simulink model "VIPR4sStEnCtrl"  (R2018b)
settings: Solver=FixedStepDiscrete  StartTime=0.0  StopTime=10.0  FixedStep=0.01  RelTol=1e-3
undefined symbols (not defined in the file or in its folder): data, KeSMSw4SSecRwRtStLgrstUpwdDnwdOpenPos1_Val, SecRwRtStBkReclnEn_Clear, SecRwRtStBkReclnEn_Set, SecRwRtStFtrstEn_Clear, SecRwRtStFtrstEn_Set, SecRwRtStFwdBkwdEn_Clear, SecRwRtStFwdBkwdEn_Set, SecRwRtStHdrstFwdBkwdEn_Clear, SecRwRtStHdrstFwdBkwdEn_Set, SecRwRtStHdrstUpwdDnwdEn_Clear, SecRwRtStHdrstUpwdDnwdEn_Set, SecRwRtStLgrstInwdOtwdEn_Clear, SecRwRtStLgrstInwdOtwdEn_Set, SecRwRtStLgrstUpwdDnwdEn_Clear, SecRwRtStLgrstUpwdDnwdEn_Set
libraries: simulink x16
settings Model: Creator=sn2xws  LastModifiedBy=sn2xws
settings Model: ModifiedHistory=|
  | 2023.11.16  V2.3.0 Issue 566045 全躺，vip，腿托打开增加前后位置
  | 2023.12.22
settings DataIOCC: SaveFormat=StructureWithTime
settings OptimizationCC: DefaultParameterBehavior=Inlined  EnhancedBackFolding=on  PassReuseOutputArgsAs=Individual arguments  ZeroExternalMemoryAtStartup=off  ZeroInternalMemoryAtStartup=off  OptimizeBlockOrder=speed  DifferentSizesBufferReuse=on  OptimizationCustomize=off
settings DebuggingCC: ParameterTunabilityLossMsg=error
settings SFSimCC: MATLABDynamicMemAlloc=off
settings RTWCC: SystemTargetFile=autosar.tlc  GenCodeOnly=on  TemplateMakefile=ert_default_tmf  Description=AUTOSAR  GenerateReport=on  IncludeHyperlinkInReport=on  LaunchReport=on  GenerateTraceInfo=on  GenerateTraceReport=on  GenerateTraceReportSl=on  GenerateTraceReportSf=on  GenerateTraceReportEml=on  GenerateCodeMetricsReport=on
settings CodeAppCC: ForceParamTrailComments=on  IgnoreCustomStorageClasses=off  OperatorAnnotations=on  SimulinkDataObjDesc=on  SFDataObjDesc=on  InsertBlockDesc=on
settings STFCustomTargetCC: TargetLangStandard=C99 (ISO)  MultiwordLength=256  ParMdlRefBuildCompliant=on  CompOptLevelCompliant=on  IncludeMdlTerminateFcn=off  CombineOutputUpdateFcns=on  SuppressErrorStatus=on  ERTCustomFileBanners=on  SupportNonFinite=off  SupportComplex=off  SupportContinuousTime=off  SupportNonInlinedSFcns=off  RemoveResetFunc=on  MATLABClassNameForMDSCustomization=Simulink.SoftwareTarget.ERTCustomization  AutosarCompliant=on  UseToolchainInfoCompliant=on  LookupTableObjectStructAxisOrder=2,1,3,4,...  LUTObjectStructOrderEvenSpacing=Size,Table,Breakpoints  SystemTargetFile=autosar.tlc
settings ERTTargetCC: TargetLangStandard=C99 (ISO)  ConcurrentExecutionCompliant=off  IncludeMdlTerminateFcn=off  SuppressErrorStatus=on  SupportNonFinite=off  SupportComplex=off  ModelStepFunctionPrototypeControlCompliant=off  CPPClassGenCompliant=off  AutosarCompliant=on  LookupTableObjectStructAxisOrder=2,1,3,4,...  LUTObjectStructOrderEvenSpacing=Size,Table,Breakpoints  InlinedParameterPlacement=NonHierarchical  ERTCustomFileTemplate=example_file_process.tlc  ERTFilePackagingFormat=Compact

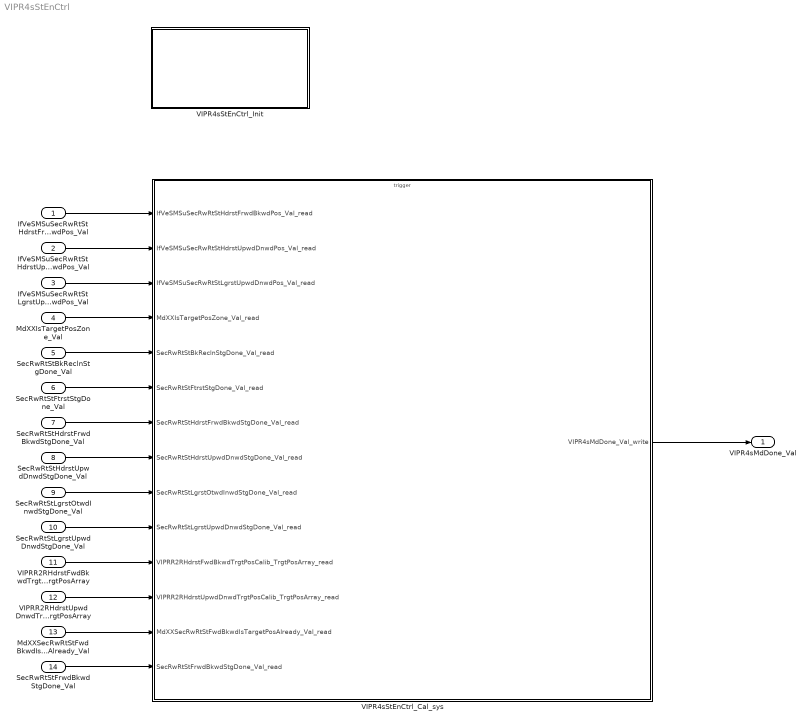
== system VIPR4sStEnCtrl ==
  IfVeSMSuSecRwRtStHdrstFrwdBkwdPos_Val : Inport  OutDataTypeStr=uint16  PortDimensions=1
  IfVeSMSuSecRwRtStHdrstUpwdDnwdPos_Val : Inport  Port=2  OutDataTypeStr=uint16  PortDimensions=1
  IfVeSMSuSecRwRtStLgrstUpwdDnwdPos_Val : Inport  Port=3  OutDataTypeStr=uint16  PortDimensions=1
  MdXXIsTargetPosZone_Val : Inport  Port=4  OutDataTypeStr=uint32  PortDimensions=1
  SecRwRtStBkReclnStgDone_Val : Inport  Port=5  OutDataTypeStr=boolean  PortDimensions=1
  SecRwRtStFtrstStgDone_Val : Inport  Port=6  OutDataTypeStr=boolean  PortDimensions=1
  SecRwRtStHdrstFrwdBkwdStgDone_Val : Inport  Port=7  OutDataTypeStr=boolean  PortDimensions=1
  SecRwRtStHdrstUpwdDnwdStgDone_Val : Inport  Port=8  OutDataTypeStr=boolean  PortDimensions=1
  SecRwRtStLgrstOtwdInwdStgDone_Val : Inport  Port=9  OutDataTypeStr=boolean  PortDimensions=1
  SecRwRtStLgrstUpwdDnwdStgDone_Val : Inport  Port=10  OutDataTypeStr=boolean  PortDimensions=1
  VIPRR2RHdrstFwdBkwdTrgtPosCalib_TrgtPosArray : Inport  Description=|  Port=11  OutDataTypeStr=uint16  PortDimensions=3
      | 0:Pos
      | 1:Max
      | 2:Min
  VIPRR2RHdrstUpwdDnwdTrgtPosCalib_TrgtPosArray : Inport  Description=|  Port=12  OutDataTypeStr=uint16  PortDimensions=3
      | 0:Pos
      | 1:Max
      | 2:Min
  MdXXSecRwRtStFwdBkwdIsTargetPosAlready_Val : Inport  Port=13  OutDataTypeStr=uint32  PortDimensions=1
  SecRwRtStFrwdBkwdStgDone_Val : Inport  Port=14  OutDataTypeStr=boolean  PortDimensions=1
  VIPR4sStEnCtrl_Cal_sys : Subsystem
  VIPR4sStEnCtrl_Init : Subsystem
  VIPR4sMdDone_Val : Outport  OutDataTypeStr=uint8  PortDimensions=1
  wires:
  IfVeSMSuSecRwRtStHdrstFrwdBkwdPos_Val/1 -> VIPR4sStEnCtrl_Cal_sys/1(IfVeSMSuSecRwRtStHdrstFrwdBkwdPos_Val_read)
  IfVeSMSuSecRwRtStHdrstUpwdDnwdPos_Val/1 -> VIPR4sStEnCtrl_Cal_sys/2(IfVeSMSuSecRwRtStHdrstUpwdDnwdPos_Val_read)
  IfVeSMSuSecRwRtStLgrstUpwdDnwdPos_Val/1 -> VIPR4sStEnCtrl_Cal_sys/3(IfVeSMSuSecRwRtStLgrstUpwdDnwdPos_Val_read)
  MdXXIsTargetPosZone_Val/1 -> VIPR4sStEnCtrl_Cal_sys/4(MdXXIsTargetPosZone_Val_read)
  SecRwRtStBkReclnStgDone_Val/1 -> VIPR4sStEnCtrl_Cal_sys/5(SecRwRtStBkReclnStgDone_Val_read)
  SecRwRtStFtrstStgDone_Val/1 -> VIPR4sStEnCtrl_Cal_sys/6(SecRwRtStFtrstStgDone_Val_read)
  SecRwRtStHdrstFrwdBkwdStgDone_Val/1 -> VIPR4sStEnCtrl_Cal_sys/7(SecRwRtStHdrstFrwdBkwdStgDone_Val_read)
  SecRwRtStHdrstUpwdDnwdStgDone_Val/1 -> VIPR4sStEnCtrl_Cal_sys/8(SecRwRtStHdrstUpwdDnwdStgDone_Val_read)
  SecRwRtStLgrstOtwdInwdStgDone_Val/1 -> VIPR4sStEnCtrl_Cal_sys/9(SecRwRtStLgrstOtwdInwdStgDone_Val_read)
  SecRwRtStLgrstUpwdDnwdStgDone_Val/1 -> VIPR4sStEnCtrl_Cal_sys/10(SecRwRtStLgrstUpwdDnwdStgDone_Val_read)
  VIPRR2RHdrstFwdBkwdTrgtPosCalib_TrgtPosArray/1 -> VIPR4sStEnCtrl_Cal_sys/11(VIPRR2RHdrstFwdBkwdTrgtPosCalib_TrgtPosArray_read)
  VIPRR2RHdrstUpwdDnwdTrgtPosCalib_TrgtPosArray/1 -> VIPR4sStEnCtrl_Cal_sys/12(VIPRR2RHdrstUpwdDnwdTrgtPosCalib_TrgtPosArray_read)
  VIPR4sStEnCtrl_Cal_sys/1(VIPR4sMdDone_Val_write) -> VIPR4sMdDone_Val/1
  MdXXSecRwRtStFwdBkwdIsTargetPosAlready_Val/1 -> VIPR4sStEnCtrl_Cal_sys/13(MdXXSecRwRtStFwdBkwdIsTargetPosAlready_Val_read)
  SecRwRtStFrwdBkwdStgDone_Val/1 -> VIPR4sStEnCtrl_Cal_sys/14(SecRwRtStFrwdBkwdStgDone_Val_read)

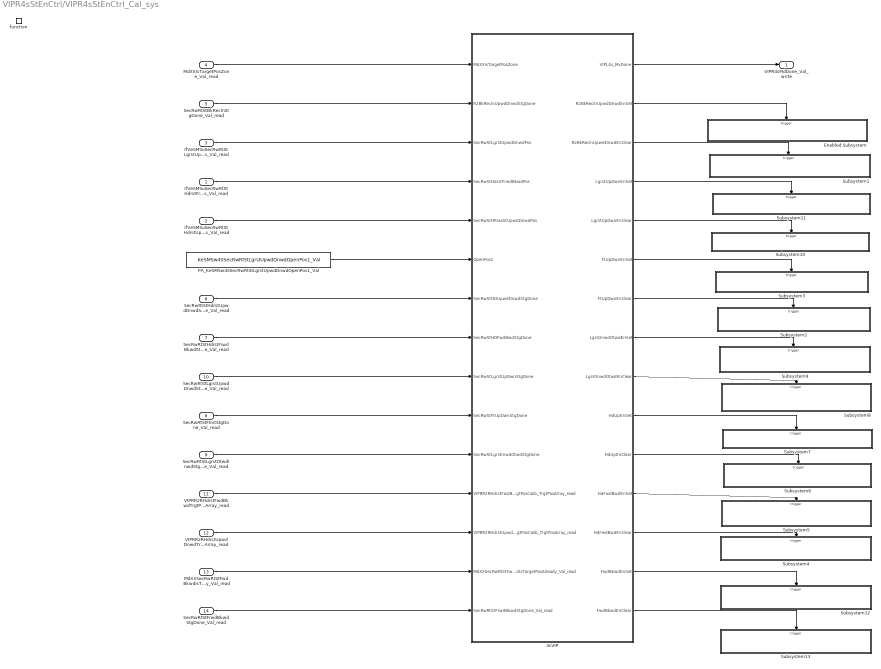
== system VIPR4sStEnCtrl/VIPR4sStEnCtrl_Cal_sys ==
  IfVeSMSuSecRwRtStHdrstFrwdBkwdPos_Val_read : Inport
  IfVeSMSuSecRwRtStHdrstUpwdDnwdPos_Val_read : Inport  Port=2
  IfVeSMSuSecRwRtStLgrstUpwdDnwdPos_Val_read : Inport  Port=3
  MdXXIsTargetPosZone_Val_read : Inport  Port=4
  SecRwRtStBkReclnStgDone_Val_read : Inport  Port=5
  SecRwRtStFtrstStgDone_Val_read : Inport  Port=6
  SecRwRtStHdrstFrwdBkwdStgDone_Val_read : Inport  Port=7
  SecRwRtStHdrstUpwdDnwdStgDone_Val_read : Inport  Port=8
  SecRwRtStLgrstOtwdInwdStgDone_Val_read : Inport  Port=9
  SecRwRtStLgrstUpwdDnwdStgDone_Val_read : Inport  Port=10
  VIPRR2RHdrstFwdBkwdTrgtPosCalib_TrgtPosArray_read : Inport  Port=11
  VIPRR2RHdrstUpwdDnwdTrgtPosCalib_TrgtPosArray_read : Inport  Port=12
  MdXXSecRwRtStFwdBkwdIsTargetPosAlready_Val_read : Inport  Port=13
  SecRwRtStFrwdBkwdStgDone_Val_read : Inport  Port=14
  function : TriggerPort  TriggerType=function-call  IsSimulinkFunction=on  FunctionName=VIPR4sStEnCtrl_Cal  VariantControl=(inherit)
  4sVIP : Subsystem
  Enabled Subsystem : Subsystem  TreatAsAtomicUnit=on
  PA_KeSMSw4SSecRwRtStLgrstUpwdDnwdOpenPos1_Val : Constant  Value=KeSMSw4SSecRwRtStLgrstUpwdDnwdOpenPos1_Val
  Subsystem1 : Subsystem
  Subsystem10 : Subsystem
  Subsystem11 : Subsystem
  Subsystem12 : Subsystem
  Subsystem13 : Subsystem
  Subsystem2 : Subsystem
  Subsystem3 : Subsystem
  Subsystem4 : Subsystem
  Subsystem5 : Subsystem
  Subsystem6 : Subsystem
  Subsystem7 : Subsystem
  Subsystem8 : Subsystem
  Subsystem9 : Subsystem
  VIPR4sMdDone_Val_write : Outport
      settings: EnsureOutportIsVirtual=on
  wires:
  IfVeSMSuSecRwRtStHdrstFrwdBkwdPos_Val_read/1 -> 4sVIP/4(SecRwStHdrstFrwdBkwdPos)
  IfVeSMSuSecRwRtStHdrstUpwdDnwdPos_Val_read/1 -> 4sVIP/5(SecRwStHPassStUpwdDnwdPos)
  VIPRR2RHdrstFwdBkwdTrgtPosCalib_TrgtPosArray_read/1 -> 4sVIP/12(VIPRR2RHdrstFwdBkwdTrgtPosCalib_TrgtPosArray_read)
  VIPRR2RHdrstUpwdDnwdTrgtPosCalib_TrgtPosArray_read/1 -> 4sVIP/13(VIPRR2RHdrstUpwdDnwdTrgtPosCalib_TrgtPosArray_read)
  4sVIP/1(VIPL4s_MvDone) -> VIPR4sMdDone_Val_write/1
  PA_KeSMSw4SSecRwRtStLgrstUpwdDnwdOpenPos1_Val/1 -> 4sVIP/6(OpenPos1)
  MdXXIsTargetPosZone_Val_read/1 -> 4sVIP/1(MdXXIsTargetPosZone)
  SecRwRtStBkReclnStgDone_Val_read/1 -> 4sVIP/2(R2BkReclnUpwdDnwdStgDone)
  IfVeSMSuSecRwRtStLgrstUpwdDnwdPos_Val_read/1 -> 4sVIP/3(SecRwStLgrstUpwdDnwdPos)
  SecRwRtStHdrstUpwdDnwdStgDone_Val_read/1 -> 4sVIP/7(SecRwStHDUpwdDnwdStgDone)
  SecRwRtStHdrstFrwdBkwdStgDone_Val_read/1 -> 4sVIP/8(SecRwStHDFwdBwdStgDone)
  SecRwRtStLgrstUpwdDnwdStgDone_Val_read/1 -> 4sVIP/9(SecRwStLgrstUpDwnStgDone)
  SecRwRtStLgrstOtwdInwdStgDone_Val_read/1 -> 4sVIP/11(SecRwStLgrstInwdOtwdStgDone)
  SecRwRtStFtrstStgDone_Val_read/1 -> 4sVIP/10(SecRwStFtUpDwnStgDone)
  4sVIP/13(HdFwdBwdEnClear) -> Subsystem4/Trigger
  4sVIP/2(R2BkReclnUpwdDnwdEnSet) -> Enabled Subsystem/Trigger
  4sVIP/3(R2BkReclnUpwdDnwdEnClear) -> Subsystem1/Trigger
  4sVIP/5(LgrstUpDwnEnClear) -> Subsystem10/Trigger
  4sVIP/11(HdUpEnClear) -> Subsystem6/Trigger
  4sVIP/10(HdUpEnSet) -> Subsystem7/Trigger
  4sVIP/8(LgrstInwdOtwdEnSet) -> Subsystem9/Trigger
  4sVIP/9(LgrstInwdOtwdEnClear) -> Subsystem8/Trigger
  4sVIP/6(FtUpDwnEnSet) -> Subsystem3/Trigger
  4sVIP/7(FtUpDwnEnClear) -> Subsystem2/Trigger
  4sVIP/12(HdFwdBwdEnSet) -> Subsystem5/Trigger
  4sVIP/4(LgrstUpDwnEnSet) -> Subsystem11/Trigger
  MdXXSecRwRtStFwdBkwdIsTargetPosAlready_Val_read/1 -> 4sVIP/14(MdXXSecRwRtStFwdBkwdIsTargetPosAlready_Val_read)
  SecRwRtStFrwdBkwdStgDone_Val_read/1 -> 4sVIP/15(SecRwRtStFrwdBkwdStgDone_Val_read)
  4sVIP/14(FwdBkwdEnSet) -> Subsystem12/Trigger
  4sVIP/15(FwdBkwdEnClear) -> Subsystem13/Trigger

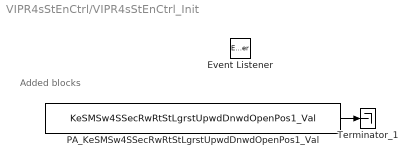
== system VIPR4sStEnCtrl/VIPR4sStEnCtrl_Init ==
  note: Added blocks
  Event Listener : EventListener  EventName=reset
  PA_KeSMSw4SSecRwRtStLgrstUpwdDnwdOpenPos1_Val : Constant  Value=KeSMSw4SSecRwRtStLgrstUpwdDnwdOpenPos1_Val
  Terminator_1 : Terminator
  wires:
  PA_KeSMSw4SSecRwRtStLgrstUpwdDnwdOpenPos1_Val/1 -> Terminator_1/1

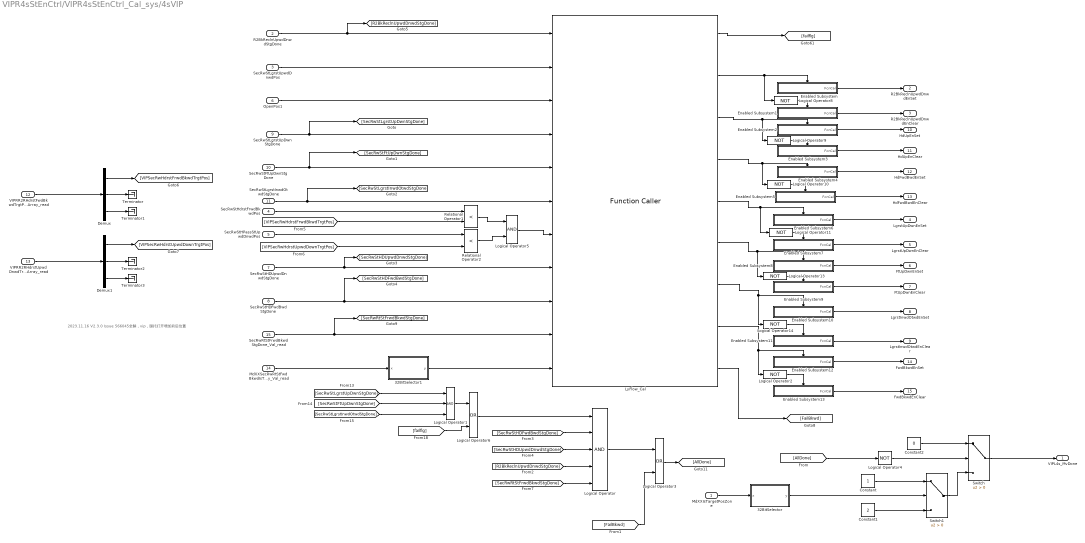
== system VIPR4sStEnCtrl/VIPR4sStEnCtrl_Cal_sys/4sVIP ==
  note: 2023.11.16 V2.3.0 Issue 566045 全躺，vip，腿托打开增加前后位置
  MdXXIsTargetPosZone : Inport
  R2BkReclnUpwdDnwdStgDone : Inport  Port=2
  SecRwStLgrstUpwdDnwdPos : Inport  Port=3
  SecRwStHdrstFrwdBkwdPos : Inport  Port=4
  SecRwStHPassStUpwdDnwdPos : Inport  Port=5
  OpenPos1 : Inport  Port=6
  SecRwStHDUpwdDnwdStgDone : Inport  Port=7
  SecRwStHDFwdBwdStgDone : Inport  Port=8
  SecRwStLgrstUpDwnStgDone : Inport  Port=9
  SecRwStFtUpDwnStgDone : Inport  Port=10
  SecRwStLgrstInwdOtwdStgDone : Inport  Port=11
  VIPRR2RHdrstFwdBkwdTrgtPosCalib_TrgtPosArray_read : Inport  Port=12
  VIPRR2RHdrstUpwdDnwdTrgtPosCalib_TrgtPosArray_read : Inport  Port=13
  MdXXSecRwRtStFwdBkwdIsTargetPosAlready_Val_read : Inport  Port=14
  SecRwRtStFrwdBkwdStgDone_Val_read : Inport  Port=15
  32BitSelector : Subsystem  mask(32 Bit Selector){BitNum=11}
      mask prompts: BitNum "Select Bit Number"
      mask help: Allows selection of a particular bit (0-31) out of a packed word up to 32 bits long. Output will be true if the bit number selected via the mask parameter is equal to one.
      mask TypeOptions BitNum: 0 | 1 | 2 | 3 | 4 | 5 | 6 | 7 | 8 | 9 | 10 | 11 | 12 | 13 | 14 | 15 | 16 | 17 | 18 | 19 | 20 | 21 | 22 | 23 | 24 | 25 | 26 | 27 | 28 | 29 | 30 | 31
      mask Display:
      | text(0.5, 0.8,'BIT','horizontalAlignment','center')
      | text(0.5, 0.5,'SELECTOR','horizontalAlignment','center')
      | text(0.5, 0.2,['-- Bit ',char(get_param(gcb,'BitNum')),' --'],'horizontalAlignment','center')
  32BitSelector1 : Subsystem  mask(32 Bit Selector){BitNum=11}
      mask prompts: BitNum "Select Bit Number"
      mask help: Allows selection of a particular bit (0-31) out of a packed word up to 32 bits long. Output will be true if the bit number selected via the mask parameter is equal to one.
      mask TypeOptions BitNum: 0 | 1 | 2 | 3 | 4 | 5 | 6 | 7 | 8 | 9 | 10 | 11 | 12 | 13 | 14 | 15 | 16 | 17 | 18 | 19 | 20 | 21 | 22 | 23 | 24 | 25 | 26 | 27 | 28 | 29 | 30 | 31
      mask Display:
      | text(0.5, 0.8,'BIT','horizontalAlignment','center')
      | text(0.5, 0.5,'SELECTOR','horizontalAlignment','center')
      | text(0.5, 0.2,['-- Bit ',char(get_param(gcb,'BitNum')),' --'],'horizontalAlignment','center')
  Constant : Constant  OutDataTypeStr=uint8
  Constant1 : Constant  Value=2  OutDataTypeStr=uint8
  Constant2 : Constant  Value=0  OutDataTypeStr=uint8
  Demux : Demux  Outputs=3
  Demux1 : Demux  Outputs=3
  Enabled Subsystem : Subsystem  TreatAsAtomicUnit=on
  Enabled Subsystem1 : Subsystem  TreatAsAtomicUnit=on
  Enabled Subsystem10 : Subsystem  TreatAsAtomicUnit=on
  Enabled Subsystem11 : Subsystem  TreatAsAtomicUnit=on
  Enabled Subsystem12 : Subsystem  TreatAsAtomicUnit=on
  Enabled Subsystem13 : Subsystem  TreatAsAtomicUnit=on
  Enabled Subsystem2 : Subsystem  TreatAsAtomicUnit=on
  Enabled Subsystem3 : Subsystem  TreatAsAtomicUnit=on
  Enabled Subsystem4 : Subsystem  TreatAsAtomicUnit=on
  Enabled Subsystem5 : Subsystem  TreatAsAtomicUnit=on
  Enabled Subsystem6 : Subsystem  TreatAsAtomicUnit=on
  Enabled Subsystem7 : Subsystem  TreatAsAtomicUnit=on
  Enabled Subsystem8 : Subsystem  TreatAsAtomicUnit=on
  Enabled Subsystem9 : Subsystem  TreatAsAtomicUnit=on
  Logical Operator : Logic  Inputs=5  AllPortsSameDT=off  OutDataTypeStr=boolean
  Logical Operator1 : Logic  Inputs=3  AllPortsSameDT=off  OutDataTypeStr=boolean
  Logical Operator{2,4,8..11,13..14} (8 alike) : Logic  Operator=NOT  AllPortsSameDT=off  OutDataTypeStr=boolean
  Logical Operator3 : Logic  Operator=OR  AllPortsSameDT=off  OutDataTypeStr=boolean
  Logical Operator5 : Logic  AllPortsSameDT=off  OutDataTypeStr=boolean
  Logical Operator6 : Logic  Operator=OR  AllPortsSameDT=off  OutDataTypeStr=boolean
  LyFlow_Cal : FunctionCaller  FunctionPrototype=[Failflg,BkReclnEn,HdrstUpwdEn,HdrstFrwdEn,LgrstUpwdDnwdEn,FtrstEn,LgrstInwdOtwdEn,FwdBkwdEn,FailBkwd] = LyFlow_Cal(BkReclnStgDone,LgrstUpwdDnwdPos,LgrstUpwdDnwdOpenPos1,LgrstUpwdStgDone,FtrstStgDone,LgrstInwdStgDone,Chkhdflg,HdrstUpwdDnwdStgDone,HdrstFrwdBkwdStgDone,FwdBkwdStgDone,FwdBkwdIsPosAlready)  InputArgumentSpecifications=boolean(true), uint16(1), uint16(1), boolean(true), boolean(true), boolean(true), boolean(true), boolean(true), boolean(true), boolean(true), boolean(true)  OutputArgumentSpecifications=boolean(true), boolean(true), boolean(true), boolean(true), boolean(true), boolean(true), boolean(true), boolean(true), boolean(true)
  Relational Operator1 : RelationalOperator  Operator=<  OutDataTypeStr=boolean  RndMeth=Simplest
  Relational Operator2 : RelationalOperator  Operator=<  OutDataTypeStr=boolean  RndMeth=Simplest
  Switch : Switch  Criteria=u2 > Threshold
  Switch1 : Switch  Criteria=u2 > Threshold
  Terminator{,1..3} (4 alike) : Terminator
  VIPL4s_MvDone : Outport
  R2BkReclnUpwdDnwdEnSet : Outport  Port=2
  R2BkReclnUpwdDnwdEnClear : Outport  Port=3
  LgrstUpDwnEnSet : Outport  Port=4
  LgrstUpDwnEnClear : Outport  Port=5
  FtUpDwnEnSet : Outport  Port=6
  FtUpDwnEnClear : Outport  Port=7
  LgrstInwdOtwdEnSet : Outport  Port=8
  LgrstInwdOtwdEnClear : Outport  Port=9
  HdUpEnSet : Outport  Port=10
  HdUpEnClear : Outport  Port=11
  HdFwdBwdEnSet : Outport  Port=12
  HdFwdBwdEnClear : Outport  Port=13
  FwdBkwdEnSet : Outport  Port=14
  FwdBkwdEnClear : Outport  Port=15
  wires:
  [VIPSecRwHdrstUpwdDownTrgtPos] -> Relational Operator2/2
  [R2BkReclnUpwdDnwdStgDone] -> Logical Operator/4
  [SecRwStFtUpDwnStgDone] -> Logical Operator1/2
  [SecRwStHDFwdBwdStgDone] -> Logical Operator/2
  SecRwStHDFwdBwdStgDone/1 -> [SecRwStHDFwdBwdStgDone], LyFlow_Cal/9
  Logical Operator5/1 -> LyFlow_Cal/7
  OpenPos1/1 -> LyFlow_Cal/3
  SecRwStLgrstInwdOtwdStgDone/1 -> [SecRwStLgrstInwdOtwdStgDone], LyFlow_Cal/6
  [failflg] -> Logical Operator6/2
  SecRwStHdrstFrwdBkwdPos/1 -> Relational Operator1/1
  Relational Operator2/1 -> Logical Operator5/2
  SecRwStFtUpDwnStgDone/1 -> LyFlow_Cal/5, [SecRwStFtUpDwnStgDone]
  [SecRwStLgrstInwdOtwdStgDone] -> Logical Operator1/3
  SecRwStHPassStUpwdDnwdPos/1 -> Relational Operator2/1
  [SecRwStLgrstUpDwnStgDone] -> Logical Operator1/1
  Logical Operator1/1 -> Logical Operator6/1
  Logical Operator6/1 -> Logical Operator/1
  [SecRwStHDUpwdDnwdStgDone] -> Logical Operator/3
  MdXXIsTargetPosZone/1 -> 32BitSelector/1(x)
  Relational Operator1/1 -> Logical Operator5/1
  SecRwStHDUpwdDnwdStgDone/1 -> [SecRwStHDUpwdDnwdStgDone], LyFlow_Cal/8
  LyFlow_Cal/1 -> [failflg]
  SecRwStLgrstUpwdDnwdPos/1 -> LyFlow_Cal/2
  R2BkReclnUpwdDnwdStgDone/1 -> [R2BkReclnUpwdDnwdStgDone], LyFlow_Cal/1
  [VIPSecRwHdrstFrwdBkwdTrgtPos] -> Relational Operator1/2
  SecRwStLgrstUpDwnStgDone/1 -> [SecRwStLgrstUpDwnStgDone], LyFlow_Cal/4
  Switch/1 -> VIPL4s_MvDone/1
  Switch1/1 -> Switch/3
  Enabled Subsystem5/1(FcnCal) -> HdFwdBwdEnClear/1
  Enabled Subsystem6/1(FcnCal) -> LgrstUpDwnEnSet/1
  Logical Operator11/1 -> Enabled Subsystem7/Enable
  Enabled Subsystem/1(FcnCal) -> R2BkReclnUpwdDnwdEnSet/1
  LyFlow_Cal/7 -> Logical Operator14/1, Enabled Subsystem10/Enable
  Enabled Subsystem3/1(FcnCal) -> HdUpEnClear/1
  Enabled Subsystem1/1(FcnCal) -> R2BkReclnUpwdDnwdEnClear/1
  Logical Operator9/1 -> Enabled Subsystem3/Enable
  Logical Operator14/1 -> Enabled Subsystem11/Enable
  Logical Operator10/1 -> Enabled Subsystem5/Enable
  LyFlow_Cal/2 -> Logical Operator8/1, Enabled Subsystem/Enable
  LyFlow_Cal/6 -> Logical Operator13/1, Enabled Subsystem8/Enable
  Enabled Subsystem10/1(FcnCal) -> LgrstInwdOtwdEnSet/1
  Logical Operator13/1 -> Enabled Subsystem9/Enable
  Enabled Subsystem11/1(FcnCal) -> LgrstInwdOtwdEnClear/1
  Logical Operator8/1 -> Enabled Subsystem1/Enable
  Enabled Subsystem2/1(FcnCal) -> HdUpEnSet/1
  LyFlow_Cal/3 -> Logical Operator9/1, Enabled Subsystem2/Enable
  Enabled Subsystem8/1(FcnCal) -> FtUpDwnEnSet/1
  Enabled Subsystem7/1(FcnCal) -> LgrstUpDwnEnClear/1
  LyFlow_Cal/5 -> Logical Operator11/1, Enabled Subsystem6/Enable
  Enabled Subsystem4/1(FcnCal) -> HdFwdBwdEnSet/1
  LyFlow_Cal/4 -> Logical Operator10/1, Enabled Subsystem4/Enable
  Enabled Subsystem9/1(FcnCal) -> FtUpDwnEnClear/1
  VIPRR2RHdrstFwdBkwdTrgtPosCalib_TrgtPosArray_read/1 -> Demux/1
  Demux/1 -> [VIPSecRwHdrstFrwdBkwdTrgtPos]
  Demux/2 -> Terminator/1
  Demux/3 -> Terminator1/1
  Demux1/3 -> Terminator3/1
  Demux1/2 -> Terminator2/1
  Demux1/1 -> [VIPSecRwHdrstUpwdDownTrgtPos]
  VIPRR2RHdrstUpwdDnwdTrgtPosCalib_TrgtPosArray_read/1 -> Demux1/1
  Constant2/1 -> Switch/1
  Constant1/1 -> Switch1/3
  Constant/1 -> Switch1/1
  [AllDone] -> Logical Operator4/1
  Logical Operator4/1 -> Switch/2
  32BitSelector/1(y) -> Switch1/2
  SecRwRtStFrwdBkwdStgDone_Val_read/1 -> [SecRwRtStFrwdBkwdStgDone], LyFlow_Cal/10
  MdXXSecRwRtStFwdBkwdIsTargetPosAlready_Val_read/1 -> 32BitSelector1/1(x)
  Enabled Subsystem13/1(FcnCal) -> FwdBkwdEnClear/1
  Enabled Subsystem12/1(FcnCal) -> FwdBkwdEnSet/1
  Logical Operator2/1 -> Enabled Subsystem13/Enable
  LyFlow_Cal/8 -> Enabled Subsystem12/Enable, Logical Operator2/1
  LyFlow_Cal/9 -> [FailBkwd]
  Logical Operator/1 -> Logical Operator3/1
  Logical Operator3/1 -> [AllDone]
  [FailBkwd] -> Logical Operator3/2
  [SecRwRtStFrwdBkwdStgDone] -> Logical Operator/5
  32BitSelector1/1(y) -> LyFlow_Cal/11

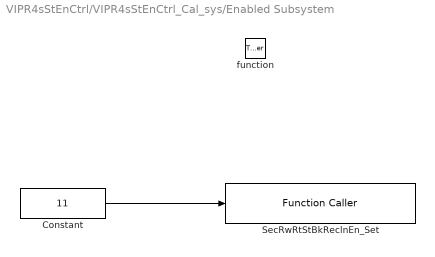
== system VIPR4sStEnCtrl/VIPR4sStEnCtrl_Cal_sys/Enabled Subsystem ==
  function : TriggerPort  TriggerType=function-call  VariantControl=Variant
  Constant : Constant  Value=11  OutDataTypeStr=uint8
  SecRwRtStBkReclnEn_Set : FunctionCaller  FunctionPrototype=SecRwRtStBkReclnEn_Set(data)  InputArgumentSpecifications=uint8(1)
  wires:
  Constant/1 -> SecRwRtStBkReclnEn_Set/1

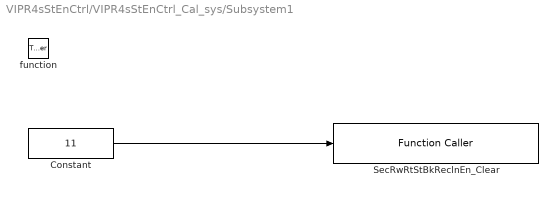
== system VIPR4sStEnCtrl/VIPR4sStEnCtrl_Cal_sys/Subsystem1 ==
  function : TriggerPort  TriggerType=function-call  VariantControl=Variant
  Constant : Constant  Value=11  OutDataTypeStr=uint8
  SecRwRtStBkReclnEn_Clear : FunctionCaller  FunctionPrototype=SecRwRtStBkReclnEn_Clear(data)  InputArgumentSpecifications=uint8(1)
  wires:
  Constant/1 -> SecRwRtStBkReclnEn_Clear/1

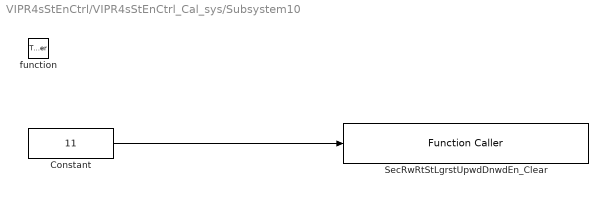
== system VIPR4sStEnCtrl/VIPR4sStEnCtrl_Cal_sys/Subsystem10 ==
  function : TriggerPort  TriggerType=function-call  VariantControl=Variant
  Constant : Constant  Value=11  OutDataTypeStr=uint8
  SecRwRtStLgrstUpwdDnwdEn_Clear : FunctionCaller  FunctionPrototype=SecRwRtStLgrstUpwdDnwdEn_Clear(data)  InputArgumentSpecifications=uint8(1)
  wires:
  Constant/1 -> SecRwRtStLgrstUpwdDnwdEn_Clear/1

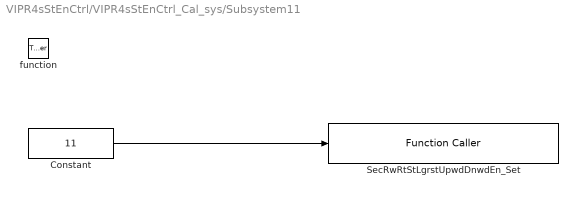
== system VIPR4sStEnCtrl/VIPR4sStEnCtrl_Cal_sys/Subsystem11 ==
  function : TriggerPort  TriggerType=function-call  VariantControl=Variant
  Constant : Constant  Value=11  OutDataTypeStr=uint8
  SecRwRtStLgrstUpwdDnwdEn_Set : FunctionCaller  FunctionPrototype=SecRwRtStLgrstUpwdDnwdEn_Set(data)  InputArgumentSpecifications=uint8(1)
  wires:
  Constant/1 -> SecRwRtStLgrstUpwdDnwdEn_Set/1

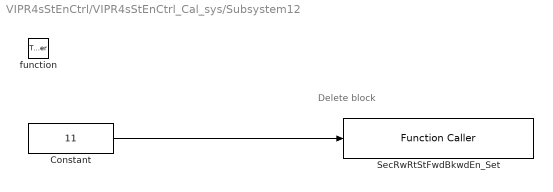
== system VIPR4sStEnCtrl/VIPR4sStEnCtrl_Cal_sys/Subsystem12 ==
  note: Delete block
  function : TriggerPort  TriggerType=function-call  VariantControl=Variant
  Constant : Constant  Value=11  OutDataTypeStr=uint8
  SecRwRtStFwdBkwdEn_Set : FunctionCaller  FunctionPrototype=SecRwRtStFwdBkwdEn_Set(data)  InputArgumentSpecifications=uint8(1)
  wires:
  Constant/1 -> SecRwRtStFwdBkwdEn_Set/1

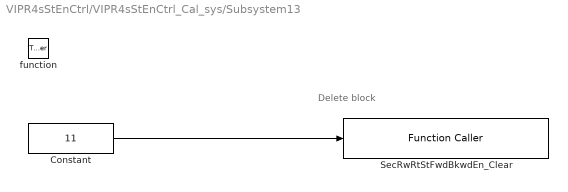
== system VIPR4sStEnCtrl/VIPR4sStEnCtrl_Cal_sys/Subsystem13 ==
  note: Delete block
  function : TriggerPort  TriggerType=function-call  VariantControl=Variant
  Constant : Constant  Value=11  OutDataTypeStr=uint8
  SecRwRtStFwdBkwdEn_Clear : FunctionCaller  FunctionPrototype=SecRwRtStFwdBkwdEn_Clear(data)  InputArgumentSpecifications=uint8(1)
  wires:
  Constant/1 -> SecRwRtStFwdBkwdEn_Clear/1

== system VIPR4sStEnCtrl/VIPR4sStEnCtrl_Cal_sys/Subsystem2 ==
  function : TriggerPort  TriggerType=function-call  VariantControl=Variant
  Constant : Constant  Value=11  OutDataTypeStr=uint8
  SecRwRtStFtrstEn_Clear : FunctionCaller  FunctionPrototype=SecRwRtStFtrstEn_Clear(data)  InputArgumentSpecifications=uint8(1)
  wires:
  Constant/1 -> SecRwRtStFtrstEn_Clear/1

== system VIPR4sStEnCtrl/VIPR4sStEnCtrl_Cal_sys/Subsystem3 ==
  function : TriggerPort  TriggerType=function-call  VariantControl=Variant
  Constant : Constant  Value=11  OutDataTypeStr=uint8
  SecRwRtStFtrstEn_Set : FunctionCaller  FunctionPrototype=SecRwRtStFtrstEn_Set(data)  InputArgumentSpecifications=uint8(1)
  wires:
  Constant/1 -> SecRwRtStFtrstEn_Set/1

== system VIPR4sStEnCtrl/VIPR4sStEnCtrl_Cal_sys/Subsystem4 ==
  function : TriggerPort  TriggerType=function-call  VariantControl=Variant
  Constant : Constant  Value=11  OutDataTypeStr=uint8
  SecRwRtStHdrstFwdBkwdEn_Clear : FunctionCaller  FunctionPrototype=SecRwRtStHdrstFwdBkwdEn_Clear(data)  InputArgumentSpecifications=uint8(1)
  wires:
  Constant/1 -> SecRwRtStHdrstFwdBkwdEn_Clear/1

== system VIPR4sStEnCtrl/VIPR4sStEnCtrl_Cal_sys/Subsystem5 ==
  function : TriggerPort  TriggerType=function-call  VariantControl=Variant
  Constant : Constant  Value=11  OutDataTypeStr=uint8
  SecRwRtStHdrstFwdBkwdEn_Set : FunctionCaller  FunctionPrototype=SecRwRtStHdrstFwdBkwdEn_Set(data)  InputArgumentSpecifications=uint8(1)
  wires:
  Constant/1 -> SecRwRtStHdrstFwdBkwdEn_Set/1

== system VIPR4sStEnCtrl/VIPR4sStEnCtrl_Cal_sys/Subsystem6 ==
  function : TriggerPort  TriggerType=function-call  VariantControl=Variant
  Constant : Constant  Value=11  OutDataTypeStr=uint8
  SecRwRtStHdrstUpwdDnwdEn_Clear : FunctionCaller  FunctionPrototype=SecRwRtStHdrstUpwdDnwdEn_Clear(data)  InputArgumentSpecifications=uint8(1)
  wires:
  Constant/1 -> SecRwRtStHdrstUpwdDnwdEn_Clear/1

== system VIPR4sStEnCtrl/VIPR4sStEnCtrl_Cal_sys/Subsystem7 ==
  function : TriggerPort  TriggerType=function-call  VariantControl=Variant
  Constant : Constant  Value=11  OutDataTypeStr=uint8
  SecRwRtStHdrstUpwdDnwdEn_Set : FunctionCaller  FunctionPrototype=SecRwRtStHdrstUpwdDnwdEn_Set(data)  InputArgumentSpecifications=uint8(1)
  wires:
  Constant/1 -> SecRwRtStHdrstUpwdDnwdEn_Set/1

== system VIPR4sStEnCtrl/VIPR4sStEnCtrl_Cal_sys/Subsystem8 ==
  function : TriggerPort  TriggerType=function-call  VariantControl=Variant
  Constant : Constant  Value=11  OutDataTypeStr=uint8
  SecRwRtStLgrstInwdOtwdEn_Clear : FunctionCaller  FunctionPrototype=SecRwRtStLgrstInwdOtwdEn_Clear(data)  InputArgumentSpecifications=uint8(1)
  wires:
  Constant/1 -> SecRwRtStLgrstInwdOtwdEn_Clear/1

== system VIPR4sStEnCtrl/VIPR4sStEnCtrl_Cal_sys/Subsystem9 ==
  function : TriggerPort  TriggerType=function-call  VariantControl=Variant
  Constant : Constant  Value=11  OutDataTypeStr=uint8
  SecRwRtStLgrstInwdOtwdEn_Set : FunctionCaller  FunctionPrototype=SecRwRtStLgrstInwdOtwdEn_Set(data)  InputArgumentSpecifications=uint8(1)
  wires:
  Constant/1 -> SecRwRtStLgrstInwdOtwdEn_Set/1

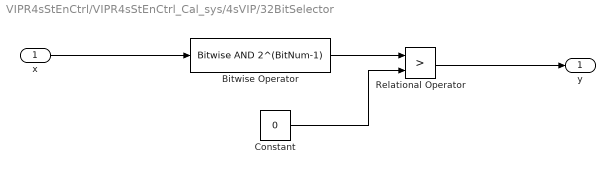
== system VIPR4sStEnCtrl/VIPR4sStEnCtrl_Cal_sys/4sVIP/32BitSelector ==
  x : Inport
  Bitwise Operator : simulink/Logic and Bit Operations/Bitwise Operator  logicop=AND  UseBitMask=on  BitMask=2^(BitNum-1)  BitMaskRealWorld=Stored Integer
  Constant : Constant  Value=0  OutDataTypeStr=uint32
  Relational Operator : RelationalOperator  Operator=>  OutDataTypeStr=boolean  RndMeth=Simplest
  y : Outport
  wires:
  Relational Operator/1 -> y/1
  Constant/1 -> Relational Operator/2
  x/1 -> Bitwise Operator/1
  Bitwise Operator/1 -> Relational Operator/1

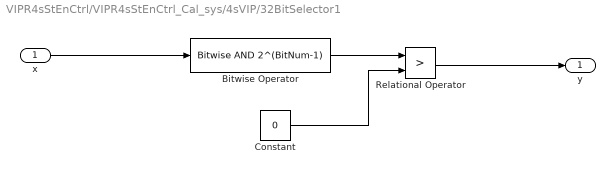
== system VIPR4sStEnCtrl/VIPR4sStEnCtrl_Cal_sys/4sVIP/32BitSelector1 ==
  x : Inport
  Bitwise Operator : simulink/Logic and Bit Operations/Bitwise Operator  logicop=AND  UseBitMask=on  BitMask=2^(BitNum-1)  BitMaskRealWorld=Stored Integer
  Constant : Constant  Value=0  OutDataTypeStr=uint32
  Relational Operator : RelationalOperator  Operator=>  OutDataTypeStr=boolean  RndMeth=Simplest
  y : Outport
  wires:
  Bitwise Operator/1 -> Relational Operator/1
  x/1 -> Bitwise Operator/1
  Constant/1 -> Relational Operator/2
  Relational Operator/1 -> y/1

== system VIPR4sStEnCtrl/VIPR4sStEnCtrl_Cal_sys/4sVIP/Enabled Subsystem ==
  Enable : EnablePort
  Function-Call Generator : simulink/Ports & Subsystems/Function-Call Generator  sample_time=-1  numberOfIterations=1
  FcnCal : Outport
  wires:
  Function-Call Generator/1 -> FcnCal/1

== system VIPR4sStEnCtrl/VIPR4sStEnCtrl_Cal_sys/4sVIP/Enabled Subsystem1 ==
  Enable : EnablePort
  Function-Call Generator : simulink/Ports & Subsystems/Function-Call Generator  sample_time=-1  numberOfIterations=1
  FcnCal : Outport
  wires:
  Function-Call Generator/1 -> FcnCal/1

== system VIPR4sStEnCtrl/VIPR4sStEnCtrl_Cal_sys/4sVIP/Enabled Subsystem10 ==
  Enable : EnablePort
  Function-Call Generator : simulink/Ports & Subsystems/Function-Call Generator  sample_time=-1  numberOfIterations=1
  FcnCal : Outport
  wires:
  Function-Call Generator/1 -> FcnCal/1

== system VIPR4sStEnCtrl/VIPR4sStEnCtrl_Cal_sys/4sVIP/Enabled Subsystem11 ==
  Enable : EnablePort
  Function-Call Generator : simulink/Ports & Subsystems/Function-Call Generator  sample_time=-1  numberOfIterations=1
  FcnCal : Outport
  wires:
  Function-Call Generator/1 -> FcnCal/1

== system VIPR4sStEnCtrl/VIPR4sStEnCtrl_Cal_sys/4sVIP/Enabled Subsystem12 ==
  Enable : EnablePort
  Function-Call Generator : simulink/Ports & Subsystems/Function-Call Generator  sample_time=-1  numberOfIterations=1
  FcnCal : Outport
  wires:
  Function-Call Generator/1 -> FcnCal/1

== system VIPR4sStEnCtrl/VIPR4sStEnCtrl_Cal_sys/4sVIP/Enabled Subsystem13 ==
  Enable : EnablePort
  Function-Call Generator : simulink/Ports & Subsystems/Function-Call Generator  sample_time=-1  numberOfIterations=1
  FcnCal : Outport
  wires:
  Function-Call Generator/1 -> FcnCal/1

== system VIPR4sStEnCtrl/VIPR4sStEnCtrl_Cal_sys/4sVIP/Enabled Subsystem2 ==
  Enable : EnablePort
  Function-Call Generator : simulink/Ports & Subsystems/Function-Call Generator  sample_time=-1  numberOfIterations=1
  FcnCal : Outport
  wires:
  Function-Call Generator/1 -> FcnCal/1

== system VIPR4sStEnCtrl/VIPR4sStEnCtrl_Cal_sys/4sVIP/Enabled Subsystem3 ==
  Enable : EnablePort
  Function-Call Generator : simulink/Ports & Subsystems/Function-Call Generator  sample_time=-1  numberOfIterations=1
  FcnCal : Outport
  wires:
  Function-Call Generator/1 -> FcnCal/1

== system VIPR4sStEnCtrl/VIPR4sStEnCtrl_Cal_sys/4sVIP/Enabled Subsystem4 ==
  Enable : EnablePort
  Function-Call Generator : simulink/Ports & Subsystems/Function-Call Generator  sample_time=-1  numberOfIterations=1
  FcnCal : Outport
  wires:
  Function-Call Generator/1 -> FcnCal/1

== system VIPR4sStEnCtrl/VIPR4sStEnCtrl_Cal_sys/4sVIP/Enabled Subsystem5 ==
  Enable : EnablePort
  Function-Call Generator : simulink/Ports & Subsystems/Function-Call Generator  sample_time=-1  numberOfIterations=1
  FcnCal : Outport
  wires:
  Function-Call Generator/1 -> FcnCal/1

== system VIPR4sStEnCtrl/VIPR4sStEnCtrl_Cal_sys/4sVIP/Enabled Subsystem6 ==
  Enable : EnablePort
  Function-Call Generator : simulink/Ports & Subsystems/Function-Call Generator  sample_time=-1  numberOfIterations=1
  FcnCal : Outport
  wires:
  Function-Call Generator/1 -> FcnCal/1

== system VIPR4sStEnCtrl/VIPR4sStEnCtrl_Cal_sys/4sVIP/Enabled Subsystem7 ==
  Enable : EnablePort
  Function-Call Generator : simulink/Ports & Subsystems/Function-Call Generator  sample_time=-1  numberOfIterations=1
  FcnCal : Outport
  wires:
  Function-Call Generator/1 -> FcnCal/1

== system VIPR4sStEnCtrl/VIPR4sStEnCtrl_Cal_sys/4sVIP/Enabled Subsystem8 ==
  Enable : EnablePort
  Function-Call Generator : simulink/Ports & Subsystems/Function-Call Generator  sample_time=-1  numberOfIterations=1
  FcnCal : Outport
  wires:
  Function-Call Generator/1 -> FcnCal/1

== system VIPR4sStEnCtrl/VIPR4sStEnCtrl_Cal_sys/4sVIP/Enabled Subsystem9 ==
  Enable : EnablePort
  Function-Call Generator : simulink/Ports & Subsystems/Function-Call Generator  sample_time=-1  numberOfIterations=1
  FcnCal : Outport
  wires:
  Function-Call Generator/1 -> FcnCal/1
